simulink model "LQG"  (R2025b)
settings: Solver=VariableStepAuto  StartTime=0.0  StopTime=20.0  RelTol=1e-3
undefined symbols (not defined in the file): A, B, C, G, K_LQR_i, K_LQR_x, Qv, Rv, Ts, xref_lqr
libraries: simulink x2, cstblocks x1
settings Model: Creator=salvo  LastModifiedBy=salvo

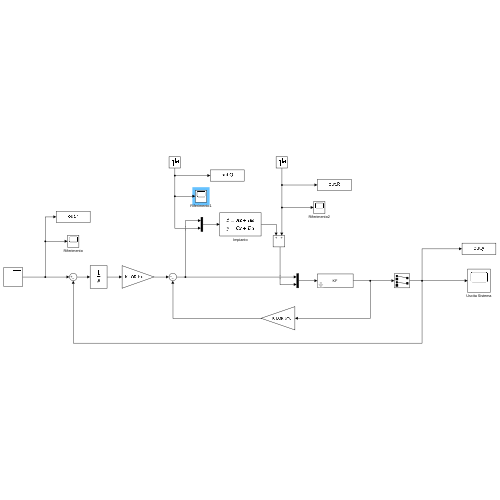
[thumbnail: Simulink's stored preview of the top-level diagram]
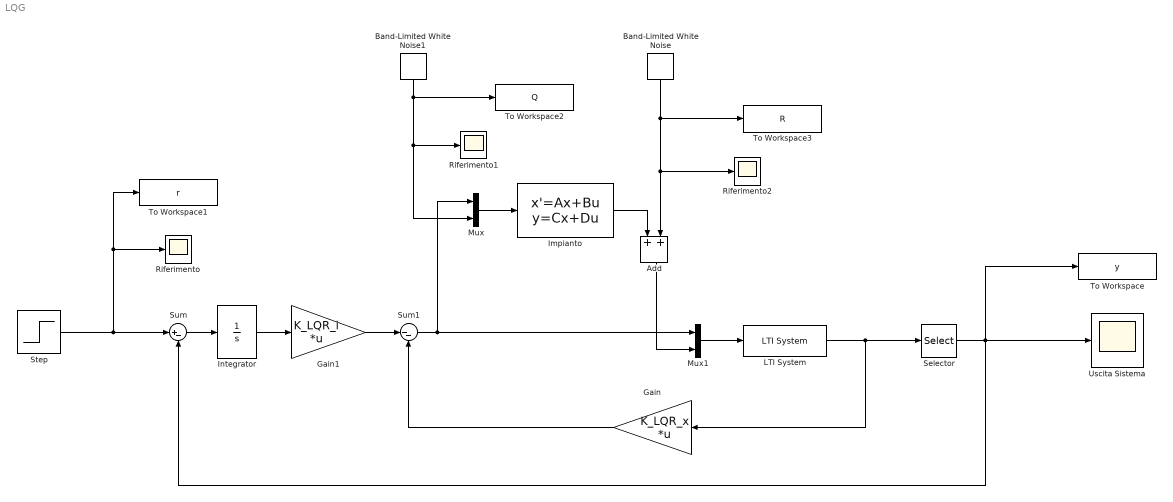
== system LQG ==
  Add : Sum
  Band-Limited White Noise : simulink/Sources/Band-Limited White Noise  Cov=diag(Rv)  Ts=Ts  seed=[23341]
  Band-Limited White Noise1 : simulink/Sources/Band-Limited White Noise  Cov=diag(Qv)  Ts=Ts  seed=[23341]
  Gain : Gain  Gain=K_LQR_x  Multiplication=Matrix(K*u)
  Gain1 : Gain  Gain=K_LQR_i  Multiplication=Matrix(K*u)
  Impianto : StateSpace  A=A  B=[B G]  C=C  D=zeros(2,6)  InitialCondition=0
  Integrator : Integrator
  LTI System : cstblocks/LTI System  sys=KF  IC=[]  PadeOrder=0
  Mux : Mux  Inputs=2
  Mux1 : Mux  Inputs=2
  Riferimento : Scope
      settings: ActiveDisplayYMinimum=-0.028675511153547856  ActiveDisplayYMaximum=0.34068834979371876  DataLoggingVariableName=ScopeData2
  Riferimento1 : Scope
      settings: ActiveDisplayYMinimum=-0.028675511153547856  ActiveDisplayYMaximum=0.34068834979371876
  Riferimento2 : Scope
      settings: ActiveDisplayYMinimum=-0.028675511153547856  ActiveDisplayYMaximum=0.34068834979371876  DataLoggingVariableName=ScopeData3
  Selector : Selector  InputPortWidth=4  IndexOptions=Index vector (dialog)  Indices=[1 3]  OutputSizes=1
  Step : Step  Time=0.0001  After=xref_lqr  SampleTime=0
  Sum : Sum  Inputs=|+-
  Sum1 : Sum  Inputs=|--
  To Workspace : ToWorkspace  VariableName=y  SaveFormat=Timeseries  SampleTime=-1
  To Workspace1 : ToWorkspace  VariableName=r  SaveFormat=Timeseries  SampleTime=-1
  To Workspace2 : ToWorkspace  VariableName=Q  SaveFormat=Timeseries  SampleTime=-1
  To Workspace3 : ToWorkspace  VariableName=R  SaveFormat=Timeseries  SampleTime=-1
  Uscita Sistema : Scope
      settings: ActiveDisplayYMinimum=-0.045828015221044481  ActiveDisplayYMaximum=0.22979707409541986
  wires:
  Integrator/1 -> Gain1/1
  Gain/1 -> Sum1/2
  Gain1/1 -> Sum1/1
  Sum/1 -> Integrator/1
  Step/1 -> Riferimento/1, To Workspace1/1, Sum/1
  Selector/1 -> To Workspace/1, Uscita Sistema/1, Sum/2
  Band-Limited White Noise/1 -> To Workspace3/1, Add/2, Riferimento2/1
  Impianto/1 -> Add/1
  Sum1/1 -> Mux/1, Mux1/1
  Band-Limited White Noise1/1 -> Mux/2, Riferimento1/1, To Workspace2/1
  Mux/1 -> Impianto/1
  Mux1/1 -> LTI System/1
  LTI System/1 -> Gain/1, Selector/1
  Add/1 -> Mux1/2
